simulink model "PLL_diff_freq"  (R2022a)
settings: Solver=FixedStepAuto  StartTime=0.0  StopTime=1  FixedStep=1/(100*fs*6)  RelTol=1e-3
values from neighbouring files (symbols this model uses):
  fs = 50*10^3    (= 50000)    [current_controller_parameters.m]
undefined symbols (not defined in the file or in its folder): I_gain_peak, I_gain_phase, P_gain_phase, RHO_MAX
libraries: simulink x2
settings Model: Creator=RTX  LastModifiedBy=RTX

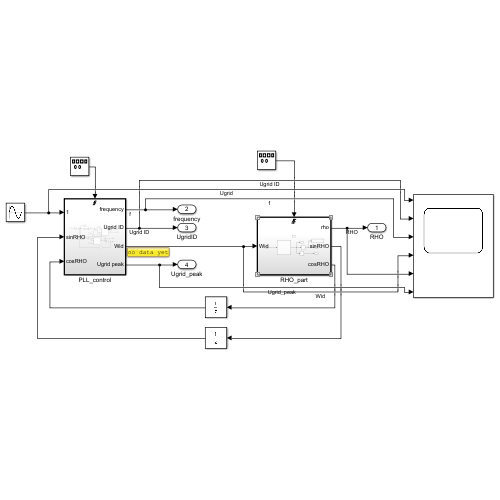
[thumbnail: Simulink's stored preview of the top-level diagram]
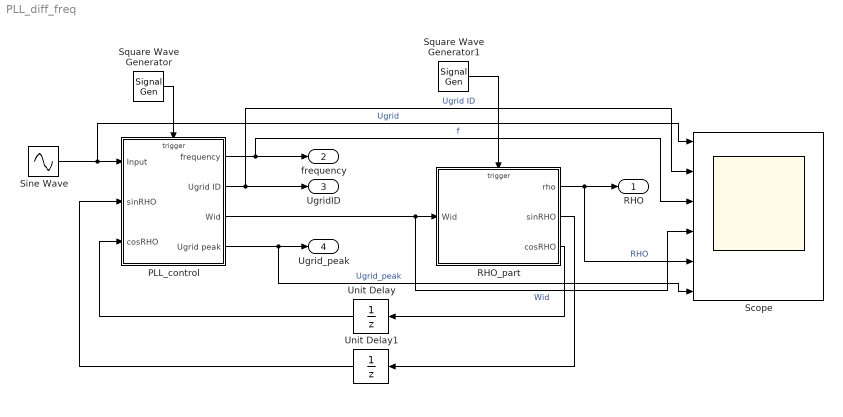
== system PLL_diff_freq ==
  PLL_control : Subsystem  TreatAsAtomicUnit=on
  RHO_part : Subsystem  TreatAsAtomicUnit=on
  Scope : Scope  NumInputPorts=6
  Sine Wave : Sin  Amplitude=48*sqrt(2)  Frequency=314.1456  Phase=1  SampleTime=0
  Square Wave Generator : SignalGenerator  WaveForm=square  Frequency=fs
  Square Wave Generator1 : SignalGenerator  WaveForm=square  Frequency=100*fs
  Unit Delay : UnitDelay  SampleTime=-1  HasFrameUpgradeWarning=on
  Unit Delay1 : UnitDelay  SampleTime=-1  HasFrameUpgradeWarning=on
  RHO : Outport
  frequency : Outport  Port=2
  UgridID : Outport  Port=3
  Ugrid_peak : Outport  Port=4
  wires:
  RHO_part/3(cosRHO) -> Unit Delay/1
  RHO_part/2(sinRHO) -> Unit Delay1/1
  RHO_part/1(rho) -> RHO/1, Scope/5  "RHO"
  Unit Delay/1 -> PLL_control/3(cosRHO)
  PLL_control/3(Wid) -> Scope/4, RHO_part/1(Wid)  "Wid"
  PLL_control/1(frequency) -> Scope/3, frequency/1  "f"
  PLL_control/2(Ugrid ID) -> Scope/2, UgridID/1  "Ugrid ID"
  PLL_control/4(Ugrid peak) -> Scope/6, Ugrid_peak/1  "Ugrid_peak"
  Sine Wave/1 -> Scope/1, PLL_control/1(Input)  "Ugrid"
  Unit Delay1/1 -> PLL_control/2(sinRHO)
  Square Wave Generator1/1 -> RHO_part/Trigger
  Square Wave Generator/1 -> PLL_control/Trigger

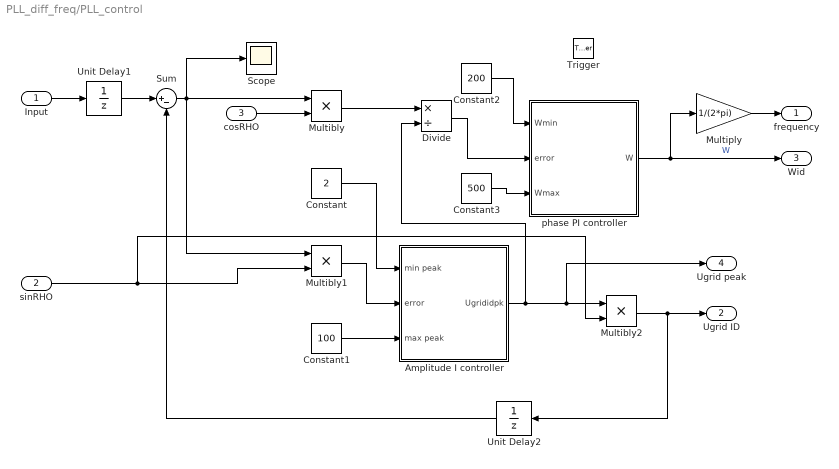
== system PLL_diff_freq/PLL_control ==
  Input : Inport
  sinRHO : Inport  Port=2
  cosRHO : Inport  Port=3
  Trigger : TriggerPort  VariantControl=(inherit)  PortDimensions=1
  Amplitude I controller : Subsystem
  Constant : Constant  Value=2
  Constant1 : Constant  Value=100
  Constant2 : Constant  Value=200
  Constant3 : Constant  Value=500
  Divide : Product  Inputs=*/
  Multibly : Product  Inputs=**
  Multibly1 : Product  Inputs=**
  Multibly2 : Product  Inputs=**
  Multiply : Gain  Gain=1/(2*pi)
  Scope : Scope
  Sum : Sum  Inputs=|+-
  Unit Delay1 : UnitDelay  SampleTime=-1  HasFrameUpgradeWarning=on
  Unit Delay2 : UnitDelay  SampleTime=-1  HasFrameUpgradeWarning=on
  phase PI controller : Subsystem
  frequency : Outport
  Ugrid ID : Outport  Port=2
  Wid : Outport  Port=3
  Ugrid peak : Outport  Port=4
  wires:
  Sum/1 -> Scope/1, Multibly/1, Multibly1/1
  Multibly/1 -> Divide/1
  Multibly1/1 -> Amplitude I controller/2(error)
  Divide/1 -> phase PI controller/2(error)
  phase PI controller/1(W) -> Multiply/1, Wid/1  "W"
  Multibly2/1 -> Ugrid ID/1, Unit Delay2/1
  Multiply/1 -> frequency/1
  Constant/1 -> Amplitude I controller/1(min peak)
  Constant1/1 -> Amplitude I controller/3(max peak)
  Constant2/1 -> phase PI controller/1(Wmin)
  Constant3/1 -> phase PI controller/3(Wmax)
  Unit Delay2/1 -> Sum/2
  Amplitude I controller/1(Ugrididpk) -> Divide/2, Multibly2/1, Ugrid peak/1
  cosRHO/1 -> Multibly/2
  sinRHO/1 -> Multibly2/2, Multibly1/2
  Input/1 -> Unit Delay1/1
  Unit Delay1/1 -> Sum/1

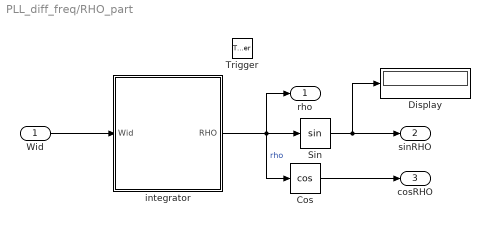
== system PLL_diff_freq/RHO_part ==
  Wid : Inport
  Trigger : TriggerPort  VariantControl=(inherit)  PortDimensions=1
  Cos : Trigonometry  Operator=cos
  Display : Display
  Sin : Trigonometry
  integrator : Subsystem
  rho : Outport
  sinRHO : Outport  Port=2
  cosRHO : Outport  Port=3
  wires:
  Cos/1 -> cosRHO/1
  Sin/1 -> sinRHO/1, Display/1
  integrator/1(RHO) -> Cos/1, Sin/1, rho/1  "rho"
  Wid/1 -> integrator/1(Wid)

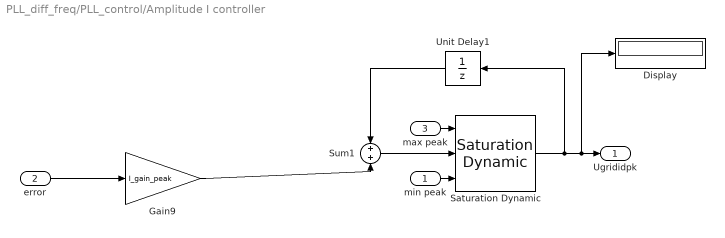
== system PLL_diff_freq/PLL_control/Amplitude I controller ==
  min peak : Inport
  error : Inport  Port=2
  max peak : Inport  Port=3
  Display : Display
  Gain9 : Gain  Gain=I_gain_peak
  Saturation Dynamic : simulink/Discontinuities/Saturation Dynamic  OutMin=[]  OutMax=[]  OutDataTypeStr=Inherit: Same as second input  OutDataType=fixdt(1, 16)  OutScaling=2^-10  DoSatur=off
  Sum1 : Sum
  Unit Delay1 : UnitDelay  InitialCondition=48*0.9*sqrt(2)  SampleTime=-1  HasFrameUpgradeWarning=on
  Ugrididpk : Outport  VectorParamsAs1DForOutWhenUnconnected=off
  wires:
  min peak/1 -> Saturation Dynamic/3
  error/1 -> Gain9/1
  Saturation Dynamic/1 -> Display/1, Ugrididpk/1, Unit Delay1/1
  Sum1/1 -> Saturation Dynamic/2
  max peak/1 -> Saturation Dynamic/1
  Gain9/1 -> Sum1/2
  Unit Delay1/1 -> Sum1/1

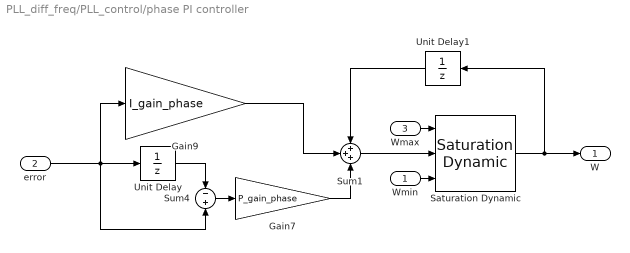
== system PLL_diff_freq/PLL_control/phase PI controller ==
  Wmin : Inport
  error : Inport  Port=2
  Wmax : Inport  Port=3
  Gain7 : Gain  Gain=P_gain_phase
  Gain9 : Gain  Gain=I_gain_phase
  Saturation Dynamic : simulink/Discontinuities/Saturation Dynamic  OutMin=[]  OutMax=[]  OutDataTypeStr=Inherit: Same as second input  OutDataType=fixdt(1, 16)  OutScaling=2^-10  DoSatur=off
  Sum1 : Sum  Inputs=+++
  Sum4 : Sum  Inputs=-|+
  Unit Delay : UnitDelay  SampleTime=-1  HasFrameUpgradeWarning=on
  Unit Delay1 : UnitDelay  InitialCondition=RHO_MAX*50*0.99  SampleTime=-1  HasFrameUpgradeWarning=on
  W : Outport  VectorParamsAs1DForOutWhenUnconnected=off
  wires:
  Unit Delay1/1 -> Sum1/1
  Unit Delay/1 -> Sum4/1
  Gain9/1 -> Sum1/2
  Wmax/1 -> Saturation Dynamic/1
  Sum4/1 -> Gain7/1
  Gain7/1 -> Sum1/3
  error/1 -> Unit Delay/1, Sum4/2, Gain9/1
  Sum1/1 -> Saturation Dynamic/2
  Saturation Dynamic/1 -> W/1, Unit Delay1/1
  Wmin/1 -> Saturation Dynamic/3

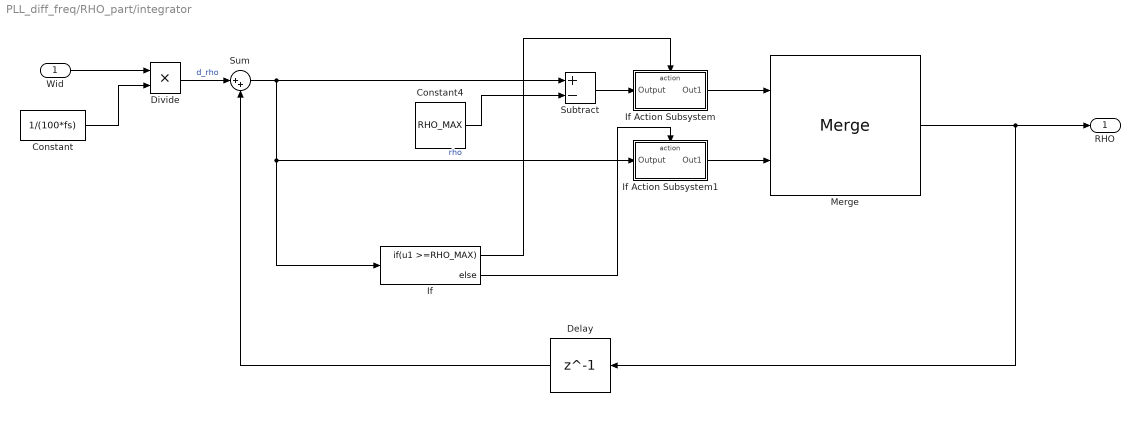
== system PLL_diff_freq/RHO_part/integrator ==
  Wid : Inport
  Constant : Constant  Value=1/(100*fs)
  Constant4 : Constant  Value=RHO_MAX
  Delay : Delay  DelayLength=1  InitialCondition=0
  Divide : Product  Inputs=**
  If : If  IfExpression=u1 >=RHO_MAX
  If Action Subsystem : Subsystem  TreatAsAtomicUnit=on
  If Action Subsystem1 : Subsystem  TreatAsAtomicUnit=on
  Merge : Merge
  Subtract : Sum  Inputs=+-
  Sum : Sum  Inputs=|++
  RHO : Outport
  wires:
  Divide/1 -> Sum/1  "d_rho"
  Delay/1 -> Sum/2
  Wid/1 -> Divide/1
  Constant/1 -> Divide/2
  If/2 -> If Action Subsystem1/Action
  If/1 -> If Action Subsystem/Action
  If Action Subsystem1/1(Out1) -> Merge/2
  Subtract/1 -> If Action Subsystem/1(Output)
  Sum/1 -> If/1, If Action Subsystem1/1(Output), Subtract/1  "rho"
  Constant4/1 -> Subtract/2
  If Action Subsystem/1(Out1) -> Merge/1
  Merge/1 -> Delay/1, RHO/1

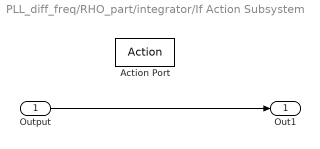
== system PLL_diff_freq/RHO_part/integrator/If Action Subsystem ==
  Output : Inport
  Action Port : ActionPort  ActionPortLabel=if(u1 >=RHO_MAX)
  Out1 : Outport
  wires:
  Output/1 -> Out1/1

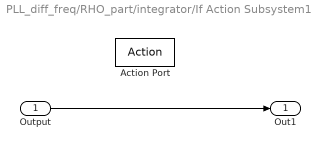
== system PLL_diff_freq/RHO_part/integrator/If Action Subsystem1 ==
  Output : Inport
  Action Port : ActionPort  ActionPortLabel=else
  Out1 : Outport
  wires:
  Output/1 -> Out1/1
